simulink model "D53_LKAS_JLU_20200911_1116"  (R2018b)
settings: Solver=ode3  StartTime=0.0  StopTime=10.0  FixedStep=0.01  RelTol=1e-3  EnableMultiTasking=on
model workspace (MAT data in the model file):
  MCOS : class17 (value not decoded)
  MCOS : class17 (value not decoded)
  MCOS : class17 (value not decoded)
  MCOS : class17 (value not decoded)
  MCOS : class17 (value not decoded)
  MCOS : class17 (value not decoded)
  MCOS : class17 (value not decoded)
  MCOS : class17 (value not decoded)
  MCOS : class17 (value not decoded)
  MCOS : class17 (value not decoded)
  MCOS : class17 (value not decoded)
  MCOS : class17 (value not decoded)
  MCOS : class17 (value not decoded)
  MCOS : class17 (value not decoded)
  MCOS : class17 (value not decoded)
  MCOS : class17 (value not decoded)
  MCOS : class17 (value not decoded)
  MCOS : class17 (value not decoded)
  MCOS : class17 (value not decoded)
  MCOS : class17 (value not decoded)
  MCOS : class17 (value not decoded)
  MCOS : class17 (value not decoded)
  MCOS : class17 (value not decoded)
  MCOS : class17 (value not decoded)
  MCOS : class17 (value not decoded)
  MCOS : class17 (value not decoded)
  MCOS : class17 (value not decoded)
  MCOS : class17 (value not decoded)
  MCOS : class17 (value not decoded)
  MCOS : class17 (value not decoded)
  MCOS : class17 (value not decoded)
  MCOS : class17 (value not decoded)
  MCOS : class17 (value not decoded)
  MCOS : class17 (value not decoded)
  MCOS : class17 (value not decoded)
  MCOS : class17 (value not decoded)
  MCOS : class17 (value not decoded)
  MCOS : class17 (value not decoded)
  MCOS : class17 (value not decoded)
  MCOS : class17 (value not decoded)
  MCOS : class17 (value not decoded)
  MCOS : class17 (value not decoded)
  MCOS : class17 (value not decoded)
  MCOS : class17 (value not decoded)
  MCOS : class17 (value not decoded)
  MCOS : class17 (value not decoded)
  MCOS : class17 (value not decoded)
  MCOS : class17 (value not decoded)
  MCOS : class17 (value not decoded)
  MCOS : class17 (value not decoded)
  MCOS : class17 (value not decoded)
  MCOS : class17 (value not decoded)
  MCOS : class17 (value not decoded)
  MCOS : class17 (value not decoded)
  MCOS : class17 (value not decoded)
  MCOS : class17 (value not decoded)
  MCOS : class17 (value not decoded)
  MCOS : class17 (value not decoded)
  MCOS : class17 (value not decoded)
  MCOS : class17 (value not decoded)
  MCOS : class17 (value not decoded)
  MCOS : class17 (value not decoded)
  MCOS : class17 (value not decoded)
  MCOS : class17 (value not decoded)
  MCOS : class17 (value not decoded)
  MCOS : class17 (value not decoded)
  MCOS : class17 (value not decoded)
  MCOS : class17 (value not decoded)
  MCOS : class17 (value not decoded)
  MCOS : class17 (value not decoded)
  MCOS : class17 (value not decoded)
  MCOS : class17 (value not decoded)
  MCOS : class17 (value not decoded)
  MCOS : class17 (value not decoded)
  MCOS : class17 (value not decoded)
  MCOS : class17 (value not decoded)
  MCOS : class17 (value not decoded)
  MCOS : class17 (value not decoded)
  MCOS : class17 (value not decoded)
  MCOS : class17 (value not decoded)
  MCOS : class17 (value not decoded)
  MCOS : class17 (value not decoded)
  MCOS : class17 (value not decoded)
  MCOS : class17 (value not decoded)
  MCOS : class17 (value not decoded)
  MCOS : class17 (value not decoded)
  MCOS : class17 (value not decoded)
  MCOS : class17 (value not decoded)
  MCOS : class17 (value not decoded)
undefined symbols (not defined in the file): LKA_CarWidth, LKA_SampleTime, LKA_StrRatio_C, LKA_Veh2CamL_C, LKA_Veh2CamW_C, LKA_WhlBaseL_C, LL_CompSWA_C, LL_CrvtPrvwT_C, LL_DesDvt_C, LL_DvtComp_C, LL_DvtPrvwT_C, LL_DvtSpdDet_vDvtSpdMin_C, LL_HdAgExT_C, LL_HdAgPrvwT_C, LL_LAccMax_C, LL_LAccRMax_C, LL_LDW_EarliestWarnLine_C, LL_LDW_LatestWarnLine_C, LL_LDWS_SUPPRESS_HEADING, LL_LFClb_TFC_DiffCtlBalance, LL_LFClb_TFC_DiffCtrlMaxSWA, LL_LFClb_TFC_DiffCtrlRatio, LL_LFClb_TFC_facmGainLutGain1_C, LL_LFClb_TFC_facmGainLutGain2_C, LL_LFClb_TFC_facmIntegRatio, LL_LFClb_TFC_facmKlat_C, LL_LFClb_TFC_FfCtlRatio_C, LL_LFClb_TFC_phiIntegCtlMaxSWA_C, LL_LFClb_TFC_tiKlatPrvwT_C, LL_LFClb_TFC_vGainLutVehSpdLwr_C, LL_LFClb_TFC_vGainLutVehSpdUpr_C, LL_LKA_EarliestWarnLine_C, LL_LKA_LatestWarnLine_C, LL_LKAExPrcs_ExitC0Dvt, LL_LKAExPrcs_ExitC0Swt, LL_LKAExPrcs_tiExitTime1, LL_LKAExPrcs_tiExitTime2, LL_LKAExPrcs_tiExitTime3, LL_LKAS_OUT_OF_CONTROL_LAT_VEL, LL_LKAS_OUT_OF_CONTROL_TTLC, LL_LKASWASyn_M0, LL_LKASWASyn_M1, LL_LKASWASyn_M2, LL_LKASWASyn_M3K, LL_LKASWASyn_SWAaddMax, LL_LKASWASyn_T2, LL_LKASWASyn_tiTrqSwaRtTime, LL_LKASWASyn_tiTrqSwaTime, LL_LKASWASyn_TrqMax, LL_LKASWASyn_TrqSwaAddSwt, LL_LKASWASyn_TrqSwaRateDiff, LL_LSpdCompT_C, LL_lStpLngth_C, LL_MAX_DELAY_EPSSTAR_TIME, LL_MAX_DRIVER_TORQUE_DISABLE, LL_MAX_DRIVER_TORQUE_ENABLE, LL_MAX_LANE_WIDTH_DISABLE, LL_MAX_LANE_WIDTH_ENABLE, LL_MAX_LAT_ACC_DISABLE, LL_MAX_LAT_ACC_ENABLE ... (+30)
libraries: simulink x134, canmsglib x52, dspstat3 x3, simulink_extras x1
(part 11 of 18)

== system D53_LKAS_JLU_20200911_1116/LL/LLOn/LKA Input Processing (LKAInP)/Predicted Heading Angle Calculation (PrHdAg)/Z Calculation (ZCalc) ==
  ZCalc_vVehSpd : Inport
  ZCalc_tiHdAgPrvwT_C : Inport  Port=2
  Divide : Product  Inputs=**  OutDataTypeStr=single
  kph to mps : Gain  Gain=1/3.6  OutDataTypeStr=single
  ZCalc_lPrvwDstZ : Outport
  wires:
  ZCalc_vVehSpd/1 -> kph to mps/1
  ZCalc_tiHdAgPrvwT_C/1 -> Divide/2
  Divide/1 -> ZCalc_lPrvwDstZ/1
  kph to mps/1 -> Divide/1

== system D53_LKAS_JLU_20200911_1116/LL/LLOn/LKA Input Processing (LKAInP)/Predicted Heading Angle Calculation (PrHdAg)/Z Calculation (ZCalc)1 ==
  ZCalc_vVehSpd : Inport
  ZCalc_tiHdAgPrvwT_C : Inport  Port=2
  Divide : Product  Inputs=**  OutDataTypeStr=single
  kph to mps : Gain  Gain=1/3.6  OutDataTypeStr=single
  ZCalc_lPrvwDstZ : Outport
  wires:
  kph to mps/1 -> Divide/1
  Divide/1 -> ZCalc_lPrvwDstZ/1
  ZCalc_tiHdAgPrvwT_C/1 -> Divide/2
  ZCalc_vVehSpd/1 -> kph to mps/1

== system D53_LKAS_JLU_20200911_1116/LL/LLOn/LKA Input Processing (LKAInP)/Previewed Curvature (PrCrvt)/Curvature Ahead of Left Lane Line (CrvtAhdLft) ==
  CrvtAhdLft_bsL0Info : Inport
  CrvtAhdLft_lPrvwDstZ : Inport  Port=2
  Add : Sum  AccumDataTypeStr=single
  Bus Selector : BusSelector  OutputSignals=L0_C2,L0_C3
  Gain : Gain  Gain=2  OutDataTypeStr=single
  Gain1 : Gain  Gain=6  OutDataTypeStr=single
  Product : Product  OutDataTypeStr=single  RndMeth=Zero
  CrvtAhdLft_crCrvtAhdLft : Outport
  wires:
  CrvtAhdLft_bsL0Info/1 -> Bus Selector/1
  Bus Selector/2 -> Gain1/1  "<L0_C3>"
  CrvtAhdLft_lPrvwDstZ/1 -> Product/2
  Bus Selector/1 -> Gain/1  "<L0_C2>"
  Gain1/1 -> Product/1
  Gain/1 -> Add/1
  Product/1 -> Add/2
  Add/1 -> CrvtAhdLft_crCrvtAhdLft/1

== system D53_LKAS_JLU_20200911_1116/LL/LLOn/LKA Input Processing (LKAInP)/Previewed Curvature (PrCrvt)/Curvature Ahead of Left Lane Line (CrvtAhdLft)1 ==
  CrvtAhdRgt_lPrvwDstZ : Inport
  CrvtAhdRgt_bsR0Info : Inport  Port=2
  Add : Sum  AccumDataTypeStr=single
  Bus Selector : BusSelector  OutputSignals=R0_C2,R0_C3
  Gain : Gain  Gain=2  OutDataTypeStr=single
  Gain1 : Gain  Gain=6  OutDataTypeStr=single
  Product : Product  OutDataTypeStr=single  RndMeth=Zero
  CrvtAhdRgt_crCrvtAhdRgt : Outport
  wires:
  CrvtAhdRgt_bsR0Info/1 -> Bus Selector/1
  Bus Selector/2 -> Gain1/1  "<R0_C3>"
  CrvtAhdRgt_lPrvwDstZ/1 -> Product/2
  Bus Selector/1 -> Gain/1  "<R0_C2>"
  Gain1/1 -> Product/1
  Gain/1 -> Add/1
  Product/1 -> Add/2
  Add/1 -> CrvtAhdRgt_crCrvtAhdRgt/1

== system D53_LKAS_JLU_20200911_1116/LL/LLOn/LKA Input Processing (LKAInP)/Previewed Curvature (PrCrvt)/Lane Information Selection (LaneInfoSel) ==
  LaneInfoSel_stLKAActvFlg : Inport
  LaneInfoSel_facmLftLane : Inport  Port=2
  LaneInfoSel_facmRgtLane : Inport  Port=3
  If : If  IfExpression=u1==1  ElseIfExpressions=u1==2
  If Action Subsystem1 : Subsystem  TreatAsAtomicUnit=on
  If Action Subsystem2 : Subsystem  TreatAsAtomicUnit=on
  If Action Subsystem3 : Subsystem  TreatAsAtomicUnit=on
  Merge : Merge  Inputs=3
  LaneInfoSel_facmActvLane : Outport
  wires:
  LaneInfoSel_facmLftLane/1 -> If Action Subsystem2/1(In1), If Action Subsystem3/1(In1)
  LaneInfoSel_facmRgtLane/1 -> If Action Subsystem1/1(In1), If Action Subsystem3/2(In2)
  LaneInfoSel_stLKAActvFlg/1 -> If/1
  If/1 -> If Action Subsystem2/Action
  If Action Subsystem2/1(Out1) -> Merge/1
  Merge/1 -> LaneInfoSel_facmActvLane/1
  If/2 -> If Action Subsystem1/Action
  If Action Subsystem1/1(Out1) -> Merge/2
  If Action Subsystem3/1(Out1) -> Merge/3
  If/3 -> If Action Subsystem3/Action

== system D53_LKAS_JLU_20200911_1116/LL/LLOn/LKA Input Processing (LKAInP)/Previewed Curvature (PrCrvt)/Z Calculation (ZCalc) ==
  ZCalc_vVehSpd : Inport
  ZCalc_tiCrvtPrvwT_C : Inport  Port=2
  Divide : Product  Inputs=**  OutDataTypeStr=single
  kph to mps : Gain  Gain=1/3.6  OutDataTypeStr=single
  ZCalc_lPrvwDstZ : Outport
  wires:
  ZCalc_vVehSpd/1 -> kph to mps/1
  ZCalc_tiCrvtPrvwT_C/1 -> Divide/2
  kph to mps/1 -> Divide/1
  Divide/1 -> ZCalc_lPrvwDstZ/1

== system D53_LKAS_JLU_20200911_1116/LL/LLOn/LKA Input Processing (LKAInP)/Steering Wheel Position Calculation (SWAPosCal)/Subsystem ==
  SWAIn : Inport
  <LKA_SampleTime> : Inport  Port=2
  Enable : EnablePort
  Constant : Constant  Value=10  OutDataTypeStr=single
  LowPass : Subsystem
  Saturation : Saturate  UpperLimit=3  LowerLimit=-3
  SWAPos : Outport  InitialOutput=0
  wires:
  Saturation/1 -> SWAPos/1
  <LKA_SampleTime>/1 -> LowPass/3(dT)
  Constant/1 -> LowPass/1(T)
  LowPass/1(y) -> Saturation/1  "SWAPos"
  SWAIn/1 -> LowPass/2(u)

== system D53_LKAS_JLU_20200911_1116/LL/LLOn/LKA Input Processing (LKAInP)/Steering Wheel Position Calculation (SWAPosCal)/Subsystem1 ==
  L0 : Inport
  R0 : Inport  Port=2
  VehSpd : Inport  Port=3
  SWA : Inport  Port=4
  Abs{2,4..7} (5 alike) : Abs
  Bus Selector : BusSelector  OutputSignals=L0_C0,L0_C1,L0_C2,L0_Q
  Bus Selector1 : BusSelector  OutputSignals=R0_C0,R0_C1,R0_C2,R0_Q
  Bus Selector2 : BusSelector  OutputSignals=LKA_SampleTime
  Compare To Constant : simulink/Logic and Bit Operations/Compare To Constant  relop===  const=3.0  OutDataTypeStr=boolean
  Compare To Constant1 : simulink/Logic and Bit Operations/Compare To Constant  relop===  const=3.0  OutDataTypeStr=boolean
  Constant : Constant  Value=0.0001  OutDataTypeStr=single
  Constant1 : Constant  Value=0.005  OutDataTypeStr=single
  Constant3 : Constant  Value=2  OutDataTypeStr=single
  Constant4 : Constant  Value=50  OutDataTypeStr=single
  Constant5 : Constant  OutDataTypeStr=single
  Divide : Product  Inputs=*/
  Logical Operator : Logic  AllPortsSameDT=off  OutDataTypeStr=boolean
  Logical Operator1 : Logic  AllPortsSameDT=off  OutDataTypeStr=boolean
  Logical Operator3 : Logic  Inputs=5  AllPortsSameDT=off  OutDataTypeStr=boolean
  Logical Operator4 : Logic  AllPortsSameDT=off  OutDataTypeStr=boolean
  Relational Operator{,1..3,7} (5 alike) : RelationalOperator  Operator=<=  OutDataTypeStr=boolean  RndMeth=Simplest
  Relational Operator6 : RelationalOperator  OutDataTypeStr=boolean  RndMeth=Simplest
  Subsystem : Subsystem
  Flg : Outport
  wires:
  Bus Selector2/1 -> Divide/2  "<LKA_SampleTime>"
  Relational Operator/1 -> Logical Operator/1
  Divide/1 -> Subsystem/2(In1)
  Bus Selector/3 -> Abs4/1  "<L0_C2>"
  Logical Operator4/1 -> Logical Operator3/3
  Bus Selector1/2 -> Abs7/1  "<R0_C1>"
  Bus Selector/2 -> Abs6/1  "<L0_C1>"
  Subsystem/1(Out) -> Flg/1
  Constant5/1 -> Relational Operator7/2
  Logical Operator/1 -> Logical Operator3/2
  SWA/1 -> Abs2/1
  Relational Operator3/1 -> Logical Operator1/2
  [LLClb_bsConstantClb] -> Bus Selector2/1
  Relational Operator1/1 -> Logical Operator/2
  Abs5/1 -> Relational Operator1/1
  Bus Selector1/3 -> Abs5/1  "<R0_C2>"
  Relational Operator7/1 -> Logical Operator3/5
  Compare To Constant/1 -> Logical Operator4/1
  Abs6/1 -> Relational Operator2/1
  Constant4/1 -> Relational Operator6/2
  VehSpd/1 -> Relational Operator6/1
  Logical Operator3/1 -> Subsystem/1(In), Subsystem/Enable  "SWA"
  Constant3/1 -> Divide/1
  Abs4/1 -> Relational Operator/1
  Constant/1 -> Relational Operator/2, Relational Operator1/2
  Constant1/1 -> Relational Operator2/2, Relational Operator3/2
  Abs7/1 -> Relational Operator3/1
  Relational Operator6/1 -> Logical Operator3/4
  Compare To Constant1/1 -> Logical Operator4/2
  Relational Operator2/1 -> Logical Operator1/1
  Bus Selector1/4 -> Compare To Constant1/1  "<R0_Q>"
  Abs2/1 -> Relational Operator7/1
  Bus Selector/4 -> Compare To Constant/1  "<L0_Q>"
  Logical Operator1/1 -> Logical Operator3/1
  R0/1 -> Bus Selector1/1
  L0/1 -> Bus Selector/1

== system D53_LKAS_JLU_20200911_1116/LL/LLOn/LKA Input Processing (LKAInP)/Under The Limit (UndrLim)/Steering Wheel Angel Max (SWAMax) ==
  SWAMax_vVehSpd : Inport
  SWAMax_aLAcc_C : Inport  Port=2
  LKA_StrRatio_C : Inport  Port=3
  LKA_WhlBaseL_C : Inport  Port=4
  Lookup Table2 : Lookup_n-D  NumberOfTableDimensions=1  BreakpointsForDimension1=[11.7,18.83,26.98,31.98,51.04,79,86.08,90.59]  BeginIndexSearchUsingPreviousIndexResult=on  Table=[0.012141,0.005179,0.00298,0.002547,0.001715,0.001283,0.001021,0.000982]  DiagnosticForOutOfRangeInput=Warning  RemoveProtectionInput=on  InternalRulePriority=Speed  OutDataTypeStr=single  InputSameDT=on
  MATLAB Function : MATLAB Function  TreatAsAtomicUnit=on
  Saturation1 : Saturate  UpperLimit=0.0117  LowerLimit=0.00237
  kph To mps : Gain  Gain=1/3.6  OutDataTypeStr=single
  SWAMax_phiSWAMax : Outport
  wires:
  MATLAB Function/1(SWAmax) -> SWAMax_phiSWAMax/1
  SWAMax_aLAcc_C/1 -> MATLAB Function/2(ax)
  Saturation1/1 -> MATLAB Function/5(K)
  Lookup Table2/1 -> Saturation1/1
  SWAMax_vVehSpd/1 -> kph To mps/1, Lookup Table2/1
  kph To mps/1 -> MATLAB Function/1(v)
  LKA_WhlBaseL_C/1 -> MATLAB Function/4(L)
  LKA_StrRatio_C/1 -> MATLAB Function/3(i)

== system D53_LKAS_JLU_20200911_1116/LL/LLOn/LKA Input Processing (LKAInP)/Under The Limit (UndrLim)/Steering Wheel Angel Rate Max (SWARMax) ==
  SWARateMax_vVehSpd : Inport
  SWARateMax_aLAccR_C : Inport  Port=2
  LKA_StrRatio_C : Inport  Port=3
  LKA_WhlBaseL_C : Inport  Port=4
  Lookup Table2 : Lookup_n-D  NumberOfTableDimensions=1  BreakpointsForDimension1=[11.7,18.83,26.98,31.98,51.04,79,86.08,90.59]  BeginIndexSearchUsingPreviousIndexResult=on  Table=[0.012141,0.005179,0.00298,0.002547,0.001715,0.001283,0.001021,0.000982]  DiagnosticForOutOfRangeInput=Warning  RemoveProtectionInput=on  InternalRulePriority=Speed  OutDataTypeStr=single  InputSameDT=on
  MATLAB Function : MATLAB Function  TreatAsAtomicUnit=on
  Saturation1 : Saturate  UpperLimit=0.0117  LowerLimit=0.00237
  kph To mps : Gain  Gain=1/3.6  OutDataTypeStr=single
  SWARMax_dphiSWARMax : Outport
  wires:
  SWARateMax_aLAccR_C/1 -> MATLAB Function/2(dax)
  Saturation1/1 -> MATLAB Function/5(K)
  Lookup Table2/1 -> Saturation1/1
  SWARateMax_vVehSpd/1 -> kph To mps/1, Lookup Table2/1
  MATLAB Function/1(SWARmax) -> SWARMax_dphiSWARMax/1
  LKA_StrRatio_C/1 -> MATLAB Function/3(i)
  LKA_WhlBaseL_C/1 -> MATLAB Function/4(L)
  kph To mps/1 -> MATLAB Function/1(v)

== system D53_LKAS_JLU_20200911_1116/LL/LLOn/LL State Determination (LLStateDet)/LL State Machine Conditions (LLSMCon)/Activation Condition (ActvC) ==
  DACMode : Inport
  InInfoSyn : Inport  Port=2
  LKAInPInfo : Inport  Port=3
  LLSMConClb : Inport  Port=4
  Activation Condition Synthesis (ActvCSyn) : Subsystem  Description=|
      | Block Name: Activation Condition Synthesis
      | Ab.: ActvCSyn
      | No.: 1.1.1.4.4
      | Rev: 0.0.1
      | Update Date: 19-3-26
  Bus Selector : BusSelector  OutputSignals=bsEPSInfo,bsVehMovInfo.ESC_VehSpd,bsLaneInfo.bsL0Info,bsLaneInfo.bsR0Info,bsLaneInfo.bsL0Info.L0_Q,bsLaneInfo.bsR0Info.R0_Q
  Bus Selector1 : BusSelector  OutputSignals=TTLC_bsTTLCInfo,Pr_bsPrInfo.bsPrHdAgInfo
  Deviation Threshold Condition (DvtThresCon) : Subsystem
  EPS Controllability Enable Condition (EPSCtlEC) : Subsystem  Description=|
      | Block Name: EPS Controllability Enable Condition
      | Ab.: EPSCtlEC
      | No.: 1.1.1.4.1
      | Rev: 0.0.1
      | Update Date: 19-3-26
  Lane Quality Enable Condition (LaneQlEC) : Subsystem  Description=|
      | Block Name: Lane Quality Enable Condition
      | Ab.: LaneQlEC
      | No.: 1.1.1.4.3
      | Rev: 0.0.1
      | Update Date: 19-3-26
  ActvC_stLDWActvCSyn : Outport
  ActvC_stLKAActvCSyn : Outport  Port=2
  wires:
  Bus Selector1/2 -> Deviation Threshold Condition (DvtThresCon)/5(DvtThresCon_bsHdAgInfo)  "<bsPrHdAgInfo>"
  Bus Selector1/1 -> Deviation Threshold Condition (DvtThresCon)/4(DvtThresCon_bsTTLCInfo)  "<TTLC_bsTTLCInfo>"
  LKAInPInfo/1 -> Bus Selector1/1
  Deviation Threshold Condition (DvtThresCon)/1(DvtThresCon_stDvtThresActvFlgLDW) -> Activation Condition Synthesis (ActvCSyn)/3(ActvCSyn_stDvtThresActvFlgLDW)
  LLSMConClb/1 -> Deviation Threshold Condition (DvtThresCon)/6(DvtThresCon_bsDvtThresClb)
  Activation Condition Synthesis (ActvCSyn)/2(ActvCSyn_stLKAActvCSyn) -> ActvC_stLKAActvCSyn/1  "ACTIVE"
  Lane Quality Enable Condition (LaneQlEC)/1(LaneQlEC_stLaneQlECFlgLKA) -> Activation Condition Synthesis (ActvCSyn)/5(ActvCSyn_stLaneQlECFlg)  "ACTIVE_LANEQUALITY"
  EPS Controllability Enable Condition (EPSCtlEC)/1(EPSCtlEC_stEPSCtlEC) -> Activation Condition Synthesis (ActvCSyn)/2(ActvCSyn_stEPSCtlEC)  "ACTIVE_EPS"
  DACMode/1 -> Activation Condition Synthesis (ActvCSyn)/1(ActvCSyn_stDACMode)
  Bus Selector/6 -> Lane Quality Enable Condition (LaneQlEC)/3(LaneQlEC_stFacmR0Ql)  "<R0_Q>"
  Bus Selector/5 -> Lane Quality Enable Condition (LaneQlEC)/2(LaneQlEC_stFacmL0Ql)  "<L0_Q>"
  Bus Selector/1 -> EPS Controllability Enable Condition (EPSCtlEC)/1(EPSCtlEC_bsEPSInfo)  "<bsEPSInfo>"
  Deviation Threshold Condition (DvtThresCon)/2(DvtThresCon_stDvtThresActvFlgLKA) -> Lane Quality Enable Condition (LaneQlEC)/1(LaneQlEC_stDvtThresActvFlg), Activation Condition Synthesis (ActvCSyn)/4(ActvCSyn_stDvtThresActvFlgLKA)
  Bus Selector/4 -> Deviation Threshold Condition (DvtThresCon)/3(DvtThresCon_bsR0Info)  "<bsR0Info>"
  Bus Selector/3 -> Deviation Threshold Condition (DvtThresCon)/2(DvtThresCon_bsL0Info)  "<bsL0Info>"
  Bus Selector/2 -> Deviation Threshold Condition (DvtThresCon)/1(DvtThresCon_vVehSpd)  "<ESC_VehSpd>"
  InInfoSyn/1 -> Bus Selector/1
  Activation Condition Synthesis (ActvCSyn)/1(ActvCSyn_stLDWActvCSyn) -> ActvC_stLDWActvCSyn/1

== system D53_LKAS_JLU_20200911_1116/LL/LLOn/LL State Determination (LLStateDet)/LL State Machine Conditions (LLSMCon)/Deactivation Condition (DeactvC) ==
  DACMode : Inport
  InInfoSyn : Inport  Port=2
  LKAInPInfo : Inport  Port=3
  LLSMConClb : Inport  Port=4
  LLState : Inport  Port=5
  ExitFlg : Inport  Port=6
  Bus Selector : BusSelector  OutputSignals=bsVehMovInfo.ESC_VehSpd,bsLaneInfo.bsL0Info,bsLaneInfo.bsR0Info,bsEPSInfo
  Bus Selector1 : BusSelector  OutputSignals=TTLC_bsTTLCInfo,Pr_bsPrInfo.bsPrHdAgInfo,Pr_bsPrInfo.bsPrCrvtInfo.crPrvwCrvt
  Deactivation Condition Synthesis (DeactvCSyn) : Subsystem  Description=|
      | Block Name: Deactivation Condition Synthesis
      | Ab.: DeactvCSyn
      | No.: 1.1.1.5.3
      | Rev: 0.0.1
      | Update Date: 19-3-26
  Deviation Threshold Condition (DvtThresCon) : Subsystem
  Driver Take Condition (DvrTkCon) : Subsystem  Description=|
      | Block Name: EPS Condition
      | Ab.: EPSC
      | No.: 1.1.1.5.2
      | Rev: 0.0.1
      | Update Date: 19-3-26
  EPS Condition (EPSC) : Subsystem  Description=|
      | Block Name: EPS Condition
      | Ab.: EPSC
      | No.: 1.1.1.5.2
      | Rev: 0.0.1
      | Update Date: 19-3-26
  DeactvC_stLDWDeactvCSyn : Outport
  DeactvC_stLKADeactvCSyn : Outport  Port=2
  wires:
  Bus Selector1/3 -> Driver Take Condition (DvrTkCon)/1(DvrTkCon_crPrvwCrvt)  "<crPrvwCrvt>"
  Bus Selector1/2 -> Deviation Threshold Condition (DvtThresCon)/5(DvtThresCon_bsHdAgInfo)  "<bsPrHdAgInfo>"
  Bus Selector1/1 -> Deviation Threshold Condition (DvtThresCon)/4(DvtThresCon_bsTTLCInfo)  "<TTLC_bsTTLCInfo>"
  LKAInPInfo/1 -> Bus Selector1/1
  Deviation Threshold Condition (DvtThresCon)/1(DvtThresCon_stDvtThresActvFlgLDW) -> Deactivation Condition Synthesis (DeactvCSyn)/2(DeactvCSyn_stDvtThresActvFlgLDW)
  Driver Take Condition (DvrTkCon)/1(DvrTkCon_stDvrTkConFlg) -> Deactivation Condition Synthesis (DeactvCSyn)/4(DvrTkCon_stDvrTkConFlg)
  Bus Selector/1 -> Deviation Threshold Condition (DvtThresCon)/1(DvtThresCon_vVehSpd), Driver Take Condition (DvrTkCon)/4(DvrTkCon_vVehSpd)  "<ESC_VehSpd>"
  Deactivation Condition Synthesis (DeactvCSyn)/2(DeactvCSyn_stLKADeactvCSyn) -> DeactvC_stLKADeactvCSyn/1  "DEACTIVE"
  DACMode/1 -> Deactivation Condition Synthesis (DeactvCSyn)/1(DeactvCSyn_stDACMode)
  ExitFlg/1 -> Deactivation Condition Synthesis (DeactvCSyn)/6(DeactvCSyn_stExitFlg)
  EPS Condition (EPSC)/1(EPSC_stEPSCFlg) -> Deactivation Condition Synthesis (DeactvCSyn)/5(DeactvCSyn_stEPSCFlg)
  Bus Selector/4 -> Driver Take Condition (DvrTkCon)/5(DvrTkCon_bsEPSInfo), EPS Condition (EPSC)/2(EPSC_bsEPSInfo)  "<bsEPSInfo>"
  LLState/1 -> EPS Condition (EPSC)/3(EPSC_bsLLState)
  Deviation Threshold Condition (DvtThresCon)/2(DvtThresCon_stDvtThresActvFlgLKA) -> Driver Take Condition (DvrTkCon)/2(DvrTkCon_stActvFlg), Deactivation Condition Synthesis (DeactvCSyn)/3(DeactvCSyn_stDvtThresActvFlgLKA)
  LLSMConClb/1 -> EPS Condition (EPSC)/1(EPSC_bsLLSMConClb), Driver Take Condition (DvrTkCon)/3(DvrTkCon_bsLLSMConClb), Deviation Threshold Condition (DvtThresCon)/6(DvtThresCon_bsDvtThresClb)
  Bus Selector/3 -> Deviation Threshold Condition (DvtThresCon)/3(DvtThresCon_bsR0Info)  "<bsR0Info>"
  Bus Selector/2 -> Deviation Threshold Condition (DvtThresCon)/2(DvtThresCon_bsL0Info)  "<bsL0Info>"
  InInfoSyn/1 -> Bus Selector/1
  Deactivation Condition Synthesis (DeactvCSyn)/1(DeactvCSyn_stLDWDeactvCSyn) -> DeactvC_stLDWDeactvCSyn/1

== system D53_LKAS_JLU_20200911_1116/LL/LLOn/LL State Determination (LLStateDet)/LL State Machine Conditions (LLSMCon)/Disable Condition (DisblC) ==
  DACMode : Inport
  InInfoSyn : Inport  Port=2
  LKAInPInfo : Inport  Port=3
  LLSMConClb : Inport  Port=4
  LLState : Inport  Port=5
  Bus Selector : BusSelector  OutputSignals=LW_LaneWidth,Pr_bsPrInfo.bsPrCrvtInfo.crPrvwCrvt,TTLC_bsTTLCInfo,Pr_bsPrInfo.bsPrDvtInfo
  Disable Condition Synthesis (DisblCSyn) : Subsystem  Description=|
      | Block Name: Disable Condition Synthesis
      | Ab.: DisblCSyn
      | No.: 1.1.1.3.8.0
      | Rev: 0.0.1
      | Update Date: 19-3-26
  Driver Intent Condition (DrvInttC) : Subsystem  Description=|
      | Block Name: Driver Intent Condition
      | Ab.: DrvInttC
      | No.: 1.1.1.3.3.0
      | Rev: 0.0.1
      | Update Date: 19-3-26
  LDW Alarm Timeout (LDWAlrmTOut) : Subsystem  Description=|
      | Block Name: LDW Alarm Timeout
      | Ab.: LDWAlrmTOut
      | No.: 1.1.1.3.6.0
      | Rev: 0.0.1
      | Update Date: 19-3-26
  LDW Own Condition (LDWOwnC) : Subsystem  Description=|
      | Block Name: LDW Own Condition
      | Ab.: LDWOwnC
      | No.: 1.1.1.3.4.0
      | Rev: 0.0.1
      | Update Date: 19-3-26
  LKA Own Condition (LKAOwnC) : Subsystem  Description=|
      | Block Name: LKA Own Condition
      | Ab.: LKAOwnC
      | No.: 1.1.1.3.5.0
      | Rev: 0.0.1
      | Update Date: 19-3-26
  Lane Condition (LaneC) : Subsystem  Description=|
      | Block Name: Lane Condition
      | Ab.: LaneC
      | No.: 1.1.1.3.2.0
      | Rev: 0.0.1
      | Update Date: 19-3-26
  Subsystem : Subsystem  Commented=on
  Vehicle State Condition (VehStateC) : Subsystem  Description=|
      | Block Name: Vehicle State Condition
      | Ab.: VehStateC
      | No.: 1.1.1.3.1.0
      | Rev: 0.0.1
      | Update Date: 19-3-26
  DisblC_stLDWDisblCSyn : Outport
  DisblC_stLKADisblCSyn : Outport  Port=2
  wires:
  Bus Selector/4 -> LDW Own Condition (LDWOwnC)/2(LDWOwnC_bsPrDvtInfo)  "<bsPrDvtInfo>"
  Bus Selector/1 -> Lane Condition (LaneC)/2(LaneC_LaneWidth)  "<LW_LaneWidth>"
  Bus Selector/2 -> Lane Condition (LaneC)/3(LaneC_crPrvwCrvt), Driver Intent Condition (DrvInttC)/3(DrvInttC_crPrvwCrvt)  "<crPrvwCrvt>"
  Bus Selector/3 -> LKA Own Condition (LKAOwnC)/3(LKAOwnC_bsTTLCInfo)  "<TTLC_bsTTLCInfo>"
  LKAInPInfo/1 -> Bus Selector/1
  Vehicle State Condition (VehStateC)/2(VehStateC) -> Subsystem/1(VehStateC)  "VehStateC"
  Lane Condition (LaneC)/2(LanCSyn) -> Subsystem/2(LanCSyn)  "LaneCSyn"
  Driver Intent Condition (DrvInttC)/2(DrvInttCSyn) -> Subsystem/3(DrvInttCSyn)  "DrvInttCSyn"
  LKA Own Condition (LKAOwnC)/2(LKAOwnC) -> Subsystem/5(LKAOwnCSyn)  "LKAOwnSyn"
  Disable Condition Synthesis (DisblCSyn)/2(DisblCSyn_stLKADisblCSyn) -> DisblC_stLKADisblCSyn/1  "DISABLE"
  InInfoSyn/1 -> Lane Condition (LaneC)/1(LaneC_bsInInfoSyn), Driver Intent Condition (DrvInttC)/1(DrvInttC_bsInInfoSyn), LKA Own Condition (LKAOwnC)/2(LKAOwnC_bsInInfoSyn), Vehicle State Condition (VehStateC)/2(VehStateC_bsInInfoSyn)
  LDW Alarm Timeout (LDWAlrmTOut)/1(LDWAlrmTOut_stLDWAlrmTOut) -> Disable Condition Synthesis (DisblCSyn)/7(DisblCSyn_stLDWAlrmTOut), Subsystem/6(LDWAlrmTOut)  "LDWAlrmTOut"
  DACMode/1 -> Disable Condition Synthesis (DisblCSyn)/1(DisblCSyn_stDACMode), LDW Own Condition (LDWOwnC)/1(LDWOwnC_stDACMode), LKA Own Condition (LKAOwnC)/1(LKAOwnC_stDACMode), Vehicle State Condition (VehStateC)/1(VehStateC_stDACMode)
  LLSMConClb/1 -> Lane Condition (LaneC)/4(LaneC_bsLLSMConClb), Driver Intent Condition (DrvInttC)/2(DrvInttC_bsLLSMConClb), LDW Own Condition (LDWOwnC)/3(LDWOwnC_bsLLSMConClb), LKA Own Condition (LKAOwnC)/5(LKAOwnC_bsLLSMConClb), LDW Alarm Timeout (LDWAlrmTOut)/2(LDWAlrmTOut_bsLLSMConClb), Vehicle State Condition (VehStateC)/3(VehStateC_bsLLSMConClb)
  LLState/1 -> LKA Own Condition (LKAOwnC)/4(LKAOwnC_bsLLState), LDW Alarm Timeout (LDWAlrmTOut)/1(LDWAlrmTOut_bsLLState)
  Disable Condition Synthesis (DisblCSyn)/1(DisblCSyn_stLDWDisblCSyn) -> DisblC_stLDWDisblCSyn/1
  LKA Own Condition (LKAOwnC)/1(LKAOwnC_stLKAOwnCSyn) -> Disable Condition Synthesis (DisblCSyn)/6(DisblCSyn_stLKAOwnC)
  LDW Own Condition (LDWOwnC)/1(LDWOwnC_stLDWOwnCSyn) -> Disable Condition Synthesis (DisblCSyn)/5(DisblCSyn_stLDWOwnC), Subsystem/4(LDWOwnCSyn)  "LDWOwnCSyn"
  Driver Intent Condition (DrvInttC)/1(DrvInttC_stDrvInttCSyn) -> Disable Condition Synthesis (DisblCSyn)/4(DisblCSyn_stDrvInttC)
  Lane Condition (LaneC)/1(LaneC_stLanCSyn) -> Disable Condition Synthesis (DisblCSyn)/3(DisblCSyn_stLaneC)
  Vehicle State Condition (VehStateC)/1(VehStateC_stVehStateCSyn) -> Disable Condition Synthesis (DisblCSyn)/2(DisblCSyn_stVehStateC)

== system D53_LKAS_JLU_20200911_1116/LL/LLOn/LL State Determination (LLStateDet)/LL State Machine Conditions (LLSMCon)/Enable Condition (EnaC) ==
  EnaC_stDACMode : Inport
  EnaC_bsInInfoSyn : Inport  Port=2
  EnaC_bsLKAInPInfo : Inport  Port=3
  EnaC_bsLLSMConClb : Inport  Port=4
  Bus Selector : BusSelector  OutputSignals=LW_LaneWidth,Pr_bsPrInfo.bsPrCrvtInfo.crPrvwCrvt,TTLC_bsTTLCInfo,Pr_bsPrInfo.bsPrDvtInfo
  Driver Intent Condition (DrvInttC) : Subsystem  Description=|
      | Block Name: Driver Intent Condition
      | Ab.: DrvInttC
      | No.: 1.1.1.2.3.0
      | Rev: 0.0.1
      | Update Date: 19-3-26
  Enable Condition Synthesis (EnaCSyn) : Subsystem  Description=|
      | Block Name: Enable Condition Synthesis
      | Ab.: EnaCSyn
      | No.: 1.1.1.2.7.0
      | Rev: 0.0.1
      | Update Date: 19-3-26
  LDW Own Condition (LDWOwnC) : Subsystem  Description=|
      | Block Name: LDW Own Condition
      | Ab.: LDWOwnC
      | No.: 1.1.1.2.4.0
      | Rev: 0.0.1
      | Update Date: 19-3-26
  LKA Own Condition (LKAOwnC) : Subsystem  Description=|
      | Block Name: LKA Own Condition
      | Ab.: LKAOwnC
      | No.: 1.1.1.2.5.0
      | Rev: 0.0.1
      | Update Date: 19-3-26
  Lane Condition (LaneC) : Subsystem  Description=|
      | Block Name: Lane Condition
      | Ab.: LaneC
      | No.: 1.1.1.2.2.0
      | Rev: 0.0.1
      | Update Date: 19-3-26
  Vehicle State Condition (VehStateC) : Subsystem  Description=|
      | Block Name: Vehicle State Condition
      | Ab.: VehStateC
      | No.: 1.1.1.2.1.0
      | Rev: 0.0.1
      | Update Date: 19-3-26
  EnaC_stLDWEnaCSyn : Outport
  EnaC_stLKAEnaCSyn : Outport  Port=2
  wires:
  Bus Selector/4 -> LDW Own Condition (LDWOwnC)/3(LDWOwnC_bsPrDvtInfo), LKA Own Condition (LKAOwnC)/6(LKAOwnC_bsPrDvtInfo)  "<bsPrDvtInfo>"
  Bus Selector/3 -> LKA Own Condition (LKAOwnC)/4(LKAOwnC_bsTTLCInfo)  "<TTLC_bsTTLCInfo>"
  Bus Selector/2 -> Lane Condition (LaneC)/3(LaneC_crPrvwCrvt)  "<crPrvwCrvt>"
  Bus Selector/1 -> Lane Condition (LaneC)/2(LaneC_LaneWidth), LKA Own Condition (LKAOwnC)/5(LKAOwnC_LaneWidth), LDW Own Condition (LDWOwnC)/2(LDWOwnC_LaneWidth)  "<LW_LaneWidth>"
  EnaC_bsLKAInPInfo/1 -> Bus Selector/1
  Enable Condition Synthesis (EnaCSyn)/2(EnaCSyn_stLKAEnaCSyn) -> EnaC_stLKAEnaCSyn/1
  EnaC_stDACMode/1 -> Enable Condition Synthesis (EnaCSyn)/1(EnaCSyn_stDACMode), LDW Own Condition (LDWOwnC)/1(LDWOwnC_stDACMode), LKA Own Condition (LKAOwnC)/1(LKAOwnC_stDACMode), Vehicle State Condition (VehStateC)/1(VehStateC_stDACMode)
  EnaC_bsLLSMConClb/1 -> Vehicle State Condition (VehStateC)/3(VehStateC_bsLLSMConClb), Lane Condition (LaneC)/4(LaneC_bsLLSMConClb), Driver Intent Condition (DrvInttC)/2(DrvInttC_bsLLSMConClb), LDW Own Condition (LDWOwnC)/4(LDWOwnC_bsLLSMConClb), LKA Own Condition (LKAOwnC)/3(LKAOwnC_bsLLSMConClb)
  Enable Condition Synthesis (EnaCSyn)/1(EnaCSyn_stLDWEnaCSyn) -> EnaC_stLDWEnaCSyn/1
  LKA Own Condition (LKAOwnC)/1(LKAOwnC_tfLKAOwnCSyn) -> Enable Condition Synthesis (EnaCSyn)/6(EnaCSyn_stLKAOwnC)
  LDW Own Condition (LDWOwnC)/1(LDWOwnC_stLDWOwnCSyn) -> Enable Condition Synthesis (EnaCSyn)/5(EnaCSyn_stLDWOwnC)
  Driver Intent Condition (DrvInttC)/1(DrvInttC_stDrvInttCSyn) -> Enable Condition Synthesis (EnaCSyn)/4(EnaCSyn_stDrvInttC)
  Lane Condition (LaneC)/1(LaneC_stLanCSyn) -> Enable Condition Synthesis (EnaCSyn)/3(EnaCSyn_stLaneC)
  Vehicle State Condition (VehStateC)/1(VehStateC_stVehStateCSyn) -> Enable Condition Synthesis (EnaCSyn)/2(EnaCSyn_stVehStateC)
  EnaC_bsInInfoSyn/1 -> Vehicle State Condition (VehStateC)/2(VehStateC_bsInInfoSyn), Lane Condition (LaneC)/1(LaneC_bsInInfoSyn), Driver Intent Condition (DrvInttC)/1(DrvInttC_bsInInfoSyn), LKA Own Condition (LKAOwnC)/2(LKAOwnC_bsInInfoSyn)

== system D53_LKAS_JLU_20200911_1116/LL/LLOn/LL State Determination (LLStateDet)/LL State Machine Conditions (LLSMCon)/Fault Condition (FaultC) ==
  FaultC_bsInInfoSyn : Inport
  FaultC_SignalFault : Inport  Port=2
  Bus Selector2 : BusSelector  OutputSignals=bsEPSInfo.EPS_LKA_State
  Bus Selector3 : BusSelector  OutputSignals=bsLaneInfo.Fusion_AdditionalInf.Carema_Status
  Bus Selector4 : BusSelector  OutputSignals=Event_FaulVehSpeed,Event_FaulSASClb,Event_FaulSASTrim,Event_FaulSWS,Event_FaulEPSLKASt,Event_FaulETATDA,Event_FaulTCUGear,Event_FaulTrqLim,Event_FaulEPSTrqSt,Event_FaulLatAcc,Event_FaulYawRate,Event_FaulLonAcc
  Bus Selector5 : BusSelector  OutputSignals=LKA_SampleTime
  Bus Selector6 : BusSelector  OutputSignals=LKAS_BSWDTC_Status,LKAS_ASWDTC_Status
  Compare To Constant{1,3..13,15..18} (16 alike) : simulink/Logic and Bit Operations/Compare To Constant  relop===  const=1  OutDataTypeStr=boolean
  Compare To Constant14 : simulink/Logic and Bit Operations/Compare To Constant  relop===  const=4  OutDataTypeStr=boolean
  Compare To Constant2 : simulink/Logic and Bit Operations/Compare To Constant  relop===  const=3  OutDataTypeStr=boolean
  Count_5s1 : Subsystem
  Count_5s2 : Subsystem
  Count_5s3 : Subsystem
  Count_5s4 : Subsystem
  Count_5s5 : Subsystem
  Demux : Demux  Outputs=16
  Logical Operator1 : Logic  Operator=OR  Inputs=9  AllPortsSameDT=off  OutDataTypeStr=boolean
  Logical Operator10 : Logic  Operator=OR  Inputs=3  AllPortsSameDT=off  OutDataTypeStr=boolean
  Logical Operator2 : Logic  Operator=OR  Inputs=4  AllPortsSameDT=off  OutDataTypeStr=boolean
  Logical Operator3 : Logic  Operator=OR  Inputs=9  AllPortsSameDT=off  OutDataTypeStr=boolean
  Logical Operator8 : Logic  Operator=OR  Inputs=4  AllPortsSameDT=off  OutDataTypeStr=boolean
  FaultC_stLDWFaultCSyn : Outport
  FaultC_stLKAFaultCSyn : Outport  Port=2
  wires:
  Bus Selector4/12 -> ?  "<Event_FaulLonAcc>"
  Bus Selector4/11 -> ?  "<Event_FaulYawRate>"
  Bus Selector4/10 -> ?  "<Event_FaulLatAcc>"
  Bus Selector4/9 -> ?  "<Event_FaulEPSTrqSt>"
  Bus Selector4/8 -> ?  "<Event_FaulTrqLim>"
  Bus Selector4/7 -> ?  "<Event_FaulTCUGear>"
  Bus Selector4/6 -> ?  "<Event_FaulETATDA>"
  Bus Selector4/5 -> ?  "<Event_FaulEPSLKASt>"
  Bus Selector4/4 -> ?  "<Event_FaulSWS>"
  Bus Selector4/3 -> ?  "<Event_FaulSASTrim>"
  Bus Selector4/2 -> ?  "<Event_FaulSASClb>"
  Bus Selector4/1 -> ?  "<Event_FaulVehSpeed>"
  Compare To Constant8/1 -> Logical Operator1/6
  Compare To Constant12/1 -> Logical Operator1/9
  [SampleTime] -> Count_5s4/1(<LKA_SampleTime>), Count_5s5/1(<LKA_SampleTime>)
  [SampleTime] -> Count_5s3/1(<LKA_SampleTime>)
  [SampleTime] -> Count_5s2/1(<LKA_SampleTime>)
  [SampleTime] -> Count_5s1/1(<LKA_SampleTime>)
  Bus Selector5/1 -> [SampleTime]  "<LKA_SampleTime>"
  Compare To Constant2/1 -> Count_5s2/Enable  "Camera_Fault"
  Bus Selector6/1 -> Demux/1  "<LKAS_BSWDTC_Status>"
  Bus Selector6/2 -> Bus Selector4/1  "<LKAS_ASWDTC_Status>"
  Count_5s3/1(Out) -> Logical Operator8/1, Logical Operator10/1  "CAN_Bus"
  Count_5s5/1(Out) -> Logical Operator8/4  "Diag_Fault"
  Count_5s4/1(Out) -> Logical Operator10/3  "Diag_Fault"
  Logical Operator3/1 -> Count_5s5/Enable
  Logical Operator2/1 -> Count_5s4/Enable, Logical Operator3/1
  Logical Operator1/1 -> Count_5s3/Enable
  FaultC_SignalFault/1 -> Bus Selector6/1
  [LLClb_bsConstantClb] -> Bus Selector5/1
  Compare To Constant11/1 -> Logical Operator1/8
  Compare To Constant9/1 -> Logical Operator1/7
  Compare To Constant6/1 -> Logical Operator1/5
  Compare To Constant5/1 -> Logical Operator1/4
  Compare To Constant4/1 -> Logical Operator1/3
  Compare To Constant3/1 -> Logical Operator1/2
  Compare To Constant1/1 -> Logical Operator1/1
  Demux/14 -> Compare To Constant16/1  "CANEve_e_BusOff_PSA1CAN"
  Demux/15 -> Compare To Constant17/1
  Demux/16 -> Compare To Constant18/1
  Demux/13 -> Compare To Constant15/1
  Demux/7 -> Compare To Constant8/1  "CANEve_e_Node_TCU_Validity"
  Demux/8 -> Compare To Constant9/1  "CANEve_e_Node_GW_Validity"
  Demux/9 -> Compare To Constant10/1  "CANEve_e_Node_Radar_Validity"
  Demux/12 -> Compare To Constant13/1
  Demux/11 -> Compare To Constant12/1  "BatteryVoltage"
  Demux/10 -> Compare To Constant11/1  "CANEve_e_Node_Camera_Validity"
  Demux/4 -> Compare To Constant5/1  "CANEve_e_Node_ESC_Validity"
  Demux/5 -> Compare To Constant6/1  "CANEve_e_Node_EPS_Validity"
  Demux/6 -> Compare To Constant7/1  "CANEve_e_Node_EMS_Validity"
  Demux/3 -> Compare To Constant4/1  "CANEve_e_Mute_PSA1CAN"
  Demux/2 -> Compare To Constant3/1  "CANEve_e_BusOff_SensorCAN"
  Demux/1 -> Compare To Constant1/1  "CANEve_e_BusOff_PSA1CAN"
  Count_5s2/1(Out) -> Logical Operator10/2, Logical Operator8/2  "Camera_Fault"
  Bus Selector3/1 -> Compare To Constant2/1  "<Carema_Status>"
  Bus Selector2/1 -> Compare To Constant14/1  "<EPS_LKA_State>"
  FaultC_bsInInfoSyn/1 -> Bus Selector2/1, Bus Selector3/1
  Logical Operator10/1 -> FaultC_stLDWFaultCSyn/1  "LDW_Fault"
  Logical Operator8/1 -> FaultC_stLKAFaultCSyn/1  "LKA_Fault"
  Count_5s1/1(Out) -> Logical Operator8/3  "EPS_Fault"
  Compare To Constant14/1 -> Count_5s1/Enable  "EPS_State_For_LKA_Fault"

== system D53_LKAS_JLU_20200911_1116/LL/LL Inputs Mapping/bsLaneInfo/LanesReconstruct /RoadSide Offset/Average Filter (AvrgFlt) ==
  In : Inport
  PtsNum : Inport  Port=2
  Add1 : Sum  AccumDataTypeStr=single  OutDataTypeStr=single
  Add2 : Sum  Inputs=-+
  Constant : Constant  OutDataTypeStr=single
  Constant1 : Constant  OutDataTypeStr=single
  Divide : Product  Inputs=**
  Divide1 : Product  Inputs=**
  Divide2 : Product  Inputs=*/
  Memory : Memory  InitialCondition=-1.75  InheritSampleTime=on
  Saturation : Saturate  UpperLimit=10000  LowerLimit=1  OutDataTypeStr=single
  Out : Outport
  wires:
  In/1 -> Divide/1
  PtsNum/1 -> Saturation/1
  Divide/1 -> Add1/1
  Constant/1 -> Add2/2
  Add2/1 -> Divide1/1
  Divide1/1 -> Add1/2
  Add1/1 -> Out/1, Memory/1
  Divide2/1 -> Add2/1, Divide/2
  Memory/1 -> Divide1/2
  Saturation/1 -> Divide2/2
  Constant1/1 -> Divide2/1

== system D53_LKAS_JLU_20200911_1116/LL/LL Inputs Mapping/bsLaneInfo/LanesReconstruct /RoadSide Offset/Average Filter (AvrgFlt)1 ==
  In : Inport
  PtsNum : Inport  Port=2
  Add1 : Sum  AccumDataTypeStr=single  OutDataTypeStr=single
  Add2 : Sum  Inputs=-+
  Constant : Constant  OutDataTypeStr=single
  Constant1 : Constant  OutDataTypeStr=single
  Divide : Product  Inputs=**
  Divide1 : Product  Inputs=**
  Divide2 : Product  Inputs=*/
  Memory : Memory  InitialCondition=1.75  InheritSampleTime=on
  Saturation : Saturate  UpperLimit=10000  LowerLimit=1  OutDataTypeStr=single
  Out : Outport
  wires:
  In/1 -> Divide/1
  PtsNum/1 -> Saturation/1
  Divide/1 -> Add1/1
  Constant/1 -> Add2/2
  Add2/1 -> Divide1/1
  Divide1/1 -> Add1/2
  Add1/1 -> Out/1, Memory/1
  Divide2/1 -> Add2/1, Divide/2
  Memory/1 -> Divide1/2
  Saturation/1 -> Divide2/2
  Constant1/1 -> Divide2/1

== system D53_LKAS_JLU_20200911_1116/LL/LL Inputs Mapping/bsLaneInfo/LanesReconstruct /RoadSide Offset/Road Width Calculation (RoadWCal) ==
  RoadWCal_L0Info : Inport
  RoadWCal_R0Info : Inport  Port=2
  Add : Sum
  Average Filter (AvrgFlt) : Subsystem
      mask Display:
      | port_label('input', 1, 'In');
      | port_label('input', 2, 'PtsNum');
      | port_label('output', 1, 'Out');
      | color('blue');
      | text(0.98,0.9,'VCDC Block','horizontalAlignment','right');
      | color('black');
      | text(0.5,0.55,'Average Filter','horizontalAlignment','center');
      | text(0.5,0.4,'(AvrgFlt)','horizontalAlignment','center');
  Bus Selector1 : BusSelector  OutputSignals=R0_C0
  Bus Selector3 : BusSelector  OutputSignals=L0_C0
  Gain : Gain  Gain=-1
  PtsNum : Constant  Value=10  OutDataTypeStr=single
  Saturation : Saturate  UpperLimit=5.5  LowerLimit=2.5
  RoadWCal_lRoadW : Outport
  wires:
  Saturation/1 -> RoadWCal_lRoadW/1
  Average Filter (AvrgFlt)/1(Out) -> Saturation/1
  Add/1 -> Average Filter (AvrgFlt)/1(In)
  PtsNum/1 -> Average Filter (AvrgFlt)/2(PtsNum)
  Gain/1 -> Add/1
  Bus Selector1/1 -> Add/2  "<R0_C0>"
  Bus Selector3/1 -> Gain/1  "<L0_C0>"
  RoadWCal_R0Info/1 -> Bus Selector1/1
  RoadWCal_L0Info/1 -> Bus Selector3/1

== system D53_LKAS_JLU_20200911_1116/LL/LLOn/LKA/Driver Torque Addition (DTA)/Subsystem/LowPass ==
  T : Inport
  u : Inport  Port=2
  dT : Inport  Port=3
  Add : Sum  Inputs=+-
  Add1 : Sum
  Add2 : Sum  OutDataTypeStr=single
  Divide : Product  Inputs=*/
  Divide1 : Product  Inputs=**
  Memory3 : Memory  InheritSampleTime=on
  SWACmdSyn_tiSmplT_C4 : Constant  OutDataTypeStr=single
  Saturation : Saturate  UpperLimit=50  LowerLimit=0
  Switch : Switch  Criteria=u2 > Threshold  Threshold=1
  Unit Delay : UnitDelay  SampleTime=-1
  y : Outport
  wires:
  T/1 -> Divide/2
  dT/1 -> Divide/1
  u/1 -> Switch/3, Add/1
  Divide/1 -> Divide1/1
  Add/1 -> Divide1/2
  Divide1/1 -> Add1/1
  Unit Delay/1 -> Add/2, Add1/2
  Add1/1 -> Switch/1
  SWACmdSyn_tiSmplT_C4/1 -> Add2/1
  Add2/1 -> Saturation/1
  Saturation/1 -> Switch/2, Memory3/1
  Memory3/1 -> Add2/2
  Switch/1 -> y/1, Unit Delay/1

== system D53_LKAS_JLU_20200911_1116/LL/LLOn/LKA/Driver Torque Addition (DTA)/Subsystem/LowPass1 ==
  T : Inport  OutDataTypeStr=single
  u : Inport  Port=2
  dT : Inport  Port=3  OutDataTypeStr=single
  Add : Sum  Inputs=+-
  Add1 : Sum
  Add2 : Sum  OutDataTypeStr=single
  Discrete Derivative : simulink/Discrete/Discrete Derivative  gainval=1.0  ICPrevScaledInput=0.0  OutMin=[]  OutMax=[]  OutDataTypeStr=single  OutputDataTypeScalingMode=single  OutDataType=fixdt(1, 16)  OutScaling=2^-10  DoSatur=off
  Divide : Product  Inputs=*/
  Divide1 : Product  Inputs=**
  Memory3 : Memory  InheritSampleTime=on
  SWACmdSyn_tiSmplT_C4 : Constant  OutDataTypeStr=single
  Saturation : Saturate  UpperLimit=50  LowerLimit=0
  Switch : Switch  Criteria=u2 > Threshold  Threshold=2
  Unit Delay : UnitDelay  SampleTime=-1
  y : Outport
  wires:
  u/1 -> Discrete Derivative/1
  Switch/1 -> Unit Delay/1, y/1
  Memory3/1 -> Add2/2
  Saturation/1 -> Memory3/1, Switch/2
  Add2/1 -> Saturation/1
  SWACmdSyn_tiSmplT_C4/1 -> Add2/1
  Add1/1 -> Switch/1
  Unit Delay/1 -> Add1/2, Add/2
  Divide1/1 -> Add1/1
  Add/1 -> Divide1/2
  Divide/1 -> Divide1/1
  Discrete Derivative/1 -> Add/1, Switch/3
  dT/1 -> Divide/1
  T/1 -> Divide/2

== system D53_LKAS_JLU_20200911_1116/LL/LLOn/LKA/Driver Torque Addition (DTA)/Subsystem1/Moving Standard Deviation2 ==
  In1 : Inport
  Delay{,1..48} (49 alike) : Delay  DelayLength=1
  Mux : Mux  Inputs=50
  Standard Deviation : dspstat3/Standard Deviation  run=off  directionMode=Entire input  dimension=2  reset_popup=None  roiEnable=off  roiType=Rectangles  roiPortion=Entire ROI  roiOutput=Individual statistics for each ROI  roiFlag=off
      settings: SourceProductName=DSP System Toolbox  SourceProductBaseCode=DS
  Out1 : Outport
  wires:
  Delay47/1 -> Mux/50
  Delay44/1 -> Delay45/1, Mux/47
  Delay45/1 -> Delay46/1, Mux/48
  Delay46/1 -> Delay47/1, Mux/49
  Delay43/1 -> Delay44/1, Mux/46
  Delay42/1 -> Delay43/1, Mux/45
  Delay39/1 -> Delay40/1, Mux/42
  Delay40/1 -> Delay41/1, Mux/43
  Delay41/1 -> Delay42/1, Mux/44
  Delay48/1 -> Delay39/1, Mux/41
  Delay38/1 -> Delay29/1, Mux/31
  Delay31/1 -> Delay32/1, Mux/34
  Delay30/1 -> Delay31/1, Mux/33
  Delay29/1 -> Delay30/1, Mux/32
  Delay32/1 -> Delay33/1, Mux/35
  Delay33/1 -> Delay34/1, Mux/36
  Delay36/1 -> Delay37/1, Mux/39
  Delay35/1 -> Delay36/1, Mux/38
  Delay34/1 -> Delay35/1, Mux/37
  Delay37/1 -> Mux/40, Delay48/1
  Delay27/1 -> Mux/30, Delay38/1
  Delay24/1 -> Delay25/1, Mux/27
  Delay25/1 -> Delay26/1, Mux/28
  Delay26/1 -> Delay27/1, Mux/29
  Delay23/1 -> Delay24/1, Mux/26
  Delay22/1 -> Delay23/1, Mux/25
  Delay19/1 -> Delay20/1, Mux/22
  Delay20/1 -> Delay21/1, Mux/23
  Delay21/1 -> Delay22/1, Mux/24
  Delay28/1 -> Delay19/1, Mux/21
  Delay9/1 -> Delay10/1, Mux/11
  Delay12/1 -> Delay13/1, Mux/14
  Delay11/1 -> Delay12/1, Mux/13
  Delay10/1 -> Delay11/1, Mux/12
  Delay13/1 -> Delay14/1, Mux/15
  Delay14/1 -> Delay15/1, Mux/16
  Delay17/1 -> Delay18/1, Mux/19
  Delay16/1 -> Delay17/1, Mux/18
  Delay15/1 -> Delay16/1, Mux/17
  Delay18/1 -> Mux/20, Delay28/1
  Delay8/1 -> Mux/10, Delay9/1
  Delay5/1 -> Delay6/1, Mux/7
  Delay6/1 -> Delay7/1, Mux/8
  Delay7/1 -> Delay8/1, Mux/9
  Delay4/1 -> Delay5/1, Mux/6
  Delay3/1 -> Delay4/1, Mux/5
  Standard Deviation/1 -> Out1/1
  Delay/1 -> Delay1/1, Mux/2
  Mux/1 -> Standard Deviation/1
  Delay1/1 -> Delay2/1, Mux/3
  Delay2/1 -> Delay3/1, Mux/4
  In1/1 -> Delay/1, Mux/1

== system D53_LKAS_JLU_20200911_1116/LL/LLOn/LKA/Driver Torque Addition (DTA)/Subsystem1/TickTime (TTime) ==
  Add2 : Sum  OutDataTypeStr=single
  Memory3 : Memory  InheritSampleTime=on
  Saturation : Saturate  UpperLimit=50  LowerLimit=0
  Out1 : Outport
  wires:
  [LKA_SampleTime] -> Add2/1
  Saturation/1 -> Memory3/1, Out1/1
  Memory3/1 -> Add2/2
  Add2/1 -> Saturation/1

== system D53_LKAS_JLU_20200911_1116/LL/LLOn/LKA/LKA Exit Processing (LKAExPrcs)/Exit Time 2/Sum Condition1 ==
  Sample Time : Inport
  Time Exit 2 : Inport  Port=2
  Enable : EnablePort  StatesWhenEnabling=reset
  Add1 : Sum  OutDataTypeStr=single
  Memory : Memory  InheritSampleTime=on
  Relational Operator : RelationalOperator  OutDataTypeStr=boolean  RndMeth=Nearest
  Saturation : Saturate  UpperLimit=10  LowerLimit=0
  Out : Outport  OutputWhenDisabled=reset  InitialOutput=0
  wires:
  Relational Operator/1 -> Out/1
  Time Exit 2/1 -> Relational Operator/2
  Sample Time/1 -> Add1/1
  Add1/1 -> Saturation/1
  Memory/1 -> Add1/2
  Saturation/1 -> Relational Operator/1, Memory/1

== system D53_LKAS_JLU_20200911_1116/LL/LLOn/LKA/LKA Exit Processing (LKAExPrcs)/Exit Time 3/Moving Standard Deviation1 ==
  In1 : Inport
  Delay{,1..48} (49 alike) : Delay  DelayLength=1
  Mux : Mux  Inputs=50
  Standard Deviation : dspstat3/Standard Deviation  run=off  directionMode=Entire input  dimension=2  reset_popup=None  roiEnable=off  roiType=Rectangles  roiPortion=Entire ROI  roiOutput=Individual statistics for each ROI  roiFlag=off
      settings: SourceProductName=DSP System Toolbox  SourceProductBaseCode=DS
  Out1 : Outport
  wires:
  In1/1 -> Mux/1, Delay/1
  Delay2/1 -> Mux/4, Delay3/1
  Delay1/1 -> Mux/3, Delay2/1
  Mux/1 -> Standard Deviation/1
  Delay/1 -> Mux/2, Delay1/1
  Standard Deviation/1 -> Out1/1
  Delay3/1 -> Mux/5, Delay4/1
  Delay4/1 -> Mux/6, Delay5/1
  Delay7/1 -> Mux/9, Delay8/1
  Delay6/1 -> Mux/8, Delay7/1
  Delay5/1 -> Mux/7, Delay6/1
  Delay8/1 -> Delay9/1, Mux/10
  Delay18/1 -> Delay28/1, Mux/20
  Delay15/1 -> Mux/17, Delay16/1
  Delay16/1 -> Mux/18, Delay17/1
  Delay17/1 -> Mux/19, Delay18/1
  Delay14/1 -> Mux/16, Delay15/1
  Delay13/1 -> Mux/15, Delay14/1
  Delay10/1 -> Mux/12, Delay11/1
  Delay11/1 -> Mux/13, Delay12/1
  Delay12/1 -> Mux/14, Delay13/1
  Delay9/1 -> Mux/11, Delay10/1
  Delay28/1 -> Mux/21, Delay19/1
  Delay21/1 -> Mux/24, Delay22/1
  Delay20/1 -> Mux/23, Delay21/1
  Delay19/1 -> Mux/22, Delay20/1
  Delay22/1 -> Mux/25, Delay23/1
  Delay23/1 -> Mux/26, Delay24/1
  Delay26/1 -> Mux/29, Delay27/1
  Delay25/1 -> Mux/28, Delay26/1
  Delay24/1 -> Mux/27, Delay25/1
  Delay27/1 -> Delay38/1, Mux/30
  Delay37/1 -> Delay48/1, Mux/40
  Delay34/1 -> Mux/37, Delay35/1
  Delay35/1 -> Mux/38, Delay36/1
  Delay36/1 -> Mux/39, Delay37/1
  Delay33/1 -> Mux/36, Delay34/1
  Delay32/1 -> Mux/35, Delay33/1
  Delay29/1 -> Mux/32, Delay30/1
  Delay30/1 -> Mux/33, Delay31/1
  Delay31/1 -> Mux/34, Delay32/1
  Delay38/1 -> Mux/31, Delay29/1
  Delay48/1 -> Mux/41, Delay39/1
  Delay41/1 -> Mux/44, Delay42/1
  Delay40/1 -> Mux/43, Delay41/1
  Delay39/1 -> Mux/42, Delay40/1
  Delay42/1 -> Mux/45, Delay43/1
  Delay43/1 -> Mux/46, Delay44/1
  Delay46/1 -> Mux/49, Delay47/1
  Delay45/1 -> Mux/48, Delay46/1
  Delay44/1 -> Mux/47, Delay45/1
  Delay47/1 -> Mux/50

== system D53_LKAS_JLU_20200911_1116/LL/LLOn/LKA/LKA Exit Processing (LKAExPrcs)/Exit Time 3/Moving Standard Deviation2 ==
  In1 : Inport
  Delay{,1..48} (49 alike) : Delay  DelayLength=1
  Mux : Mux  Inputs=50
  Standard Deviation : dspstat3/Standard Deviation  run=off  directionMode=Entire input  dimension=2  reset_popup=None  roiEnable=off  roiType=Rectangles  roiPortion=Entire ROI  roiOutput=Individual statistics for each ROI  roiFlag=off
      settings: SourceProductName=DSP System Toolbox  SourceProductBaseCode=DS
  Out1 : Outport
  wires:
  Delay47/1 -> Mux/50
  Delay44/1 -> Delay45/1, Mux/47
  Delay45/1 -> Delay46/1, Mux/48
  Delay46/1 -> Delay47/1, Mux/49
  Delay43/1 -> Delay44/1, Mux/46
  Delay42/1 -> Delay43/1, Mux/45
  Delay39/1 -> Delay40/1, Mux/42
  Delay40/1 -> Delay41/1, Mux/43
  Delay41/1 -> Delay42/1, Mux/44
  Delay48/1 -> Delay39/1, Mux/41
  Delay38/1 -> Delay29/1, Mux/31
  Delay31/1 -> Delay32/1, Mux/34
  Delay30/1 -> Delay31/1, Mux/33
  Delay29/1 -> Delay30/1, Mux/32
  Delay32/1 -> Delay33/1, Mux/35
  Delay33/1 -> Delay34/1, Mux/36
  Delay36/1 -> Delay37/1, Mux/39
  Delay35/1 -> Delay36/1, Mux/38
  Delay34/1 -> Delay35/1, Mux/37
  Delay37/1 -> Mux/40, Delay48/1
  Delay27/1 -> Mux/30, Delay38/1
  Delay24/1 -> Delay25/1, Mux/27
  Delay25/1 -> Delay26/1, Mux/28
  Delay26/1 -> Delay27/1, Mux/29
  Delay23/1 -> Delay24/1, Mux/26
  Delay22/1 -> Delay23/1, Mux/25
  Delay19/1 -> Delay20/1, Mux/22
  Delay20/1 -> Delay21/1, Mux/23
  Delay21/1 -> Delay22/1, Mux/24
  Delay28/1 -> Delay19/1, Mux/21
  Delay9/1 -> Delay10/1, Mux/11
  Delay12/1 -> Delay13/1, Mux/14
  Delay11/1 -> Delay12/1, Mux/13
  Delay10/1 -> Delay11/1, Mux/12
  Delay13/1 -> Delay14/1, Mux/15
  Delay14/1 -> Delay15/1, Mux/16
  Delay17/1 -> Delay18/1, Mux/19
  Delay16/1 -> Delay17/1, Mux/18
  Delay15/1 -> Delay16/1, Mux/17
  Delay18/1 -> Mux/20, Delay28/1
  Delay8/1 -> Mux/10, Delay9/1
  Delay5/1 -> Delay6/1, Mux/7
  Delay6/1 -> Delay7/1, Mux/8
  Delay7/1 -> Delay8/1, Mux/9
  Delay4/1 -> Delay5/1, Mux/6
  Delay3/1 -> Delay4/1, Mux/5
  Standard Deviation/1 -> Out1/1
  Delay/1 -> Delay1/1, Mux/2
  Mux/1 -> Standard Deviation/1
  Delay1/1 -> Delay2/1, Mux/3
  Delay2/1 -> Delay3/1, Mux/4
  In1/1 -> Delay/1, Mux/1

== system D53_LKAS_JLU_20200911_1116/LL/LLOn/LKA/LKA Exit Processing (LKAExPrcs)/Exit Time 3/Sum Condition ==
  In : Inport
  In1 : Inport  Port=2
  Enable : EnablePort  StatesWhenEnabling=reset
  Add1 : Sum  OutDataTypeStr=single
  Data Type Conversion : DataTypeConversion  OutDataTypeStr=uint16
  Memory : Memory  InheritSampleTime=on
  Relational Operator : RelationalOperator  OutDataTypeStr=boolean  RndMeth=Nearest
  Saturation : Saturate  UpperLimit=100000  LowerLimit=0
  Out : Outport  OutputWhenDisabled=reset  InitialOutput=0
  wires:
  Data Type Conversion/1 -> Out/1
  In1/1 -> Relational Operator/2
  In/1 -> Add1/1
  Add1/1 -> Saturation/1
  Memory/1 -> Add1/2
  Relational Operator/1 -> Data Type Conversion/1
  Saturation/1 -> Relational Operator/1, Memory/1

== system D53_LKAS_JLU_20200911_1116/LL/LLOn/LKA/LKA Exit Processing (LKAExPrcs)/Exit Time 3/Sum Condition1 ==
  In : Inport
  In1 : Inport  Port=2
  Enable : EnablePort  StatesWhenEnabling=reset
  Add1 : Sum  OutDataTypeStr=single
  Data Type Conversion : DataTypeConversion  OutDataTypeStr=uint16
  Memory : Memory  InheritSampleTime=on
  Relational Operator : RelationalOperator  OutDataTypeStr=boolean  RndMeth=Nearest
  Saturation : Saturate  UpperLimit=100000  LowerLimit=0
  Out : Outport  OutputWhenDisabled=reset  InitialOutput=0
  wires:
  Saturation/1 -> Memory/1, Relational Operator/1
  Relational Operator/1 -> Data Type Conversion/1
  Memory/1 -> Add1/2
  Add1/1 -> Saturation/1
  In/1 -> Add1/1
  In1/1 -> Relational Operator/2
  Data Type Conversion/1 -> Out/1
